simulink model "proportionalValveHarness"  (R2022b)
settings: Solver=VariableStepAuto  StartTime=0.0  StopTime=15  RelTol=1e-3  AbsTol=1e-3
libraries: fl_lib x6, nesl_utility x3, VentilatorLibrary x1
settings Model: Creator=agonzale  LastModifiedBy=fedformi_new
settings SolverCC: AutoScaleAbsTol=off  AlgebraicLoopSolver=TrustRegion
settings DebuggingCC: UnconnectedInputMsg=warning  UnconnectedOutputMsg=warning  UnconnectedLineMsg=warning  SymbolicDimsDataTypeCodeGenerationDiagnostic=none  SFMachineParentedDataDiag=warning
settings ModelReferenceCC: EnableRefExpFcnMdlSchedulingChecks=on
settings SFSimCC: CustomCodeUndefinedFunction=UseInterfaceOnly
settings SimscapeCC: SimscapeLogType=all  SimscapeLogSimulationStatistics=on  SimscapeLogLimitData=off  SimscapeLogDataHistory=10000

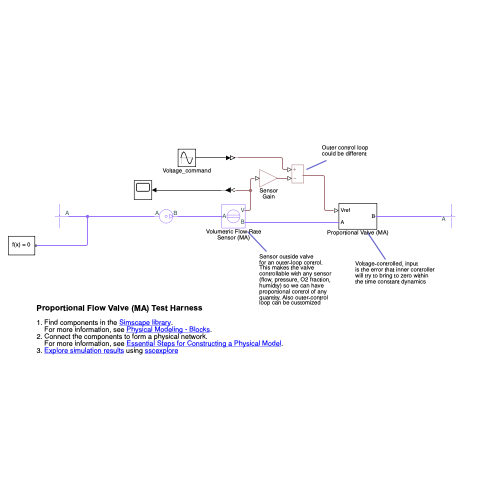
[thumbnail: Simulink's stored preview of the top-level diagram]
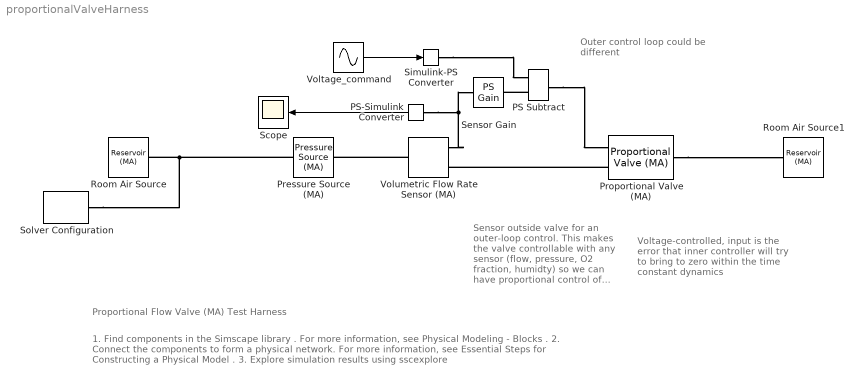
== system proportionalValveHarness ==
  note: Outer control loop
      | could be different
  note: Sensor outside valve
      | for an outer-loop control.
      | This makes the valve
      | controllable with any sensor
      | (flow, pressure, O2 fraction,
      | humidty) so we can have
      | proportional control of any
      | quantity. Also outer-control
      | loop can be customized
  note: Voltage-controlled, input
      | is the error that inner controller
      | will try to bring to zero within
      | the time constant dynamics
  note: 1. Find components in the Simscape library .
      | For more information, see Physical Modeling - Blocks .
      | 2. Connect the components to form a physical network.
      | For more information, see Essential Steps for Constructing a Physical Model .
      | 3. Explore simulation results using sscexplore
  note: Proportional Flow Valve (MA) Test Harness
  PS Subtract : fl_lib/Physical Signals/Functions/PS Subtract
  PS-Simulink Converter : nesl_utility/PS-Simulink Converter  PhysicalDomain=network_engine_domain  SubClassName=ps_output  LeftPortType=input  RightPortType=output  PseudoPeriodic=off  Frequencies=[]  VectorFormat=1-D array  Unit=lpm  AffineConversion=off
  Pressure Source (MA) : fl_lib/Moist Air/Sources/Pressure Source (MA)  power_spec=foundation.enum.power_spec.isentropic  pressure_differential=101 psi  area_A=pi*0.3^2/4 in^2  area_B=pi*0.3^2/4 in^2
      settings: InternalSimscapePortConfiguration="{\"Bottom\":[],\"Left\":[{\"id\":\"A\",\"label\":\"A\",\"type\":\"foundation.moist_air.moist_air\"}],\"Right\":[{\"id\":\"B\",\"label\":\"B\",\"type\":\"foundation.moist_air.moist_air\"}],\"Top\":[]}"
  Proportional Valve (MA) : VentilatorLibrary/Proportional Valve (MA)  D_max=0.125  area_leak=1e-5  area_A=pi*0.3^2/4  Cd=0.7  pr=0.999  area_init=1e-5  tau=0.1  Vmax=5
  Room Air Source : fl_lib/Moist Air/Elements/Reservoir (MA)  pressure_spec=foundation.enum.pressure_spec.atmospheric  reservoir_pressure=0.101325 MPa  temperature_spec=foundation.enum.temperature_spec.specified  reservoir_temperature=293 K  moisture_spec=foundation.enum.moisture_spec.relative_humidity  reservoir_RH=0.1  reservoir_x_w=0.01  reservoir_y_w=0.01  reservoir_HR=0.01  trace_gas_spec=foundation.enum.trace_gas_spec.mass_fraction  reservoir_x_g=0  reservoir_y_g=0.001  RH_ws=1  area_A=pi*0.3^2/4 in^2
  Room Air Source1 : fl_lib/Moist Air/Elements/Reservoir (MA)  pressure_spec=foundation.enum.pressure_spec.atmospheric  reservoir_pressure=0.101325 MPa  temperature_spec=foundation.enum.temperature_spec.specified  reservoir_temperature=25 degC  moisture_spec=foundation.enum.moisture_spec.relative_humidity  reservoir_RH=0.05  reservoir_x_w=0.01  reservoir_y_w=0.01  reservoir_HR=0.01  trace_gas_spec=foundation.enum.trace_gas_spec.mass_fraction  reservoir_x_g=0  reservoir_y_g=0.001  RH_ws=1  area_A=pi*0.3^2/4 in^2
  Scope : Scope
  Sensor Gain : fl_lib/Physical Signals/Functions/PS Gain  gain=5/500 V/lpm
  Simulink-PS Converter : nesl_utility/Simulink-PS Converter  PhysicalDomain=network_engine_domain  SubClassName=ps_input  LeftPortType=input  RightPortType=output  PseudoPeriodic=off  Frequencies=[]  NoiseDistribution=none  NoiseParameters=[]  Unit=V  AffineConversion=off  FilteringAndDerivatives=provide  SimscapeFilterOrder=1  InputFilterTimeConstant=0.001  UdotUserProvided=0
  Solver Configuration : nesl_utility/Solver Configuration  PhysicalDomain=network_engine_domain  SubClassName=solver  LeftPortType=input  RightPortType=generic  Tones=[]  Harmonics=[]  SimulateNoise=off  Profile=off  UseLocalSampling=off  EnableSwitchedLinearOptims=on  FrequencyDomain=off  UseCCode=off  RelTol=0.001  AbsTol=1e-06  MinStep=1e-09  ToWorkspace=off  RevertToSquareIcSolve=off  NumHomotopyIterations=100  PhasorMode=off  PhasorModeNumHarmonics=1  ConsistencySolver=NEWTON_XTOL_AFTER_FTOL  IndexReductionMethod=DerivativeReplacement  DoDC=off  ResidualTolerance=1e-09  ConsistencyTolSource=GLOBAL  ConsistencyAbsTol=0.001  ConsistencyRelTol=0.001  ConsistencyTolFactor=0.001  UseLocalSolver=off  LocalSolverChoice=NE_BACKWARD_EULER_ADVANCER  ResolveIndetEquations=on  FunctionEvalNumThread=1  LocalSolverSampleTime=1e-3  DoFixedCost=off  MaxNonlinIter=3  MaxModeIter=2  ComputeImpulses=off  ImpulseIterations=2  LinearAlgebra=auto  LinearAlgebraNumThread=0  EquationFormulation=NE_TIME_EF  DelaysMemoryBudget=1024  AutomaticFiltering=on  FilteringTimeConstant=0.001  PartitionStorageMethod=AS_NEEDED  PartitionMemoryBudget=1024  PartitionMethod=ROBUST
  Voltage_command : Sin  Amplitude=10  Frequency=2*pi/5  SampleTime=0
  Volumetric Flow Rate Sensor (MA) : fl_lib/Moist Air/Sensors/Volumetric Flow Rate Sensor (MA)  volumetric_flow_conditions=foundation.enum.volumetric_flow_conditions.standard  p_std=1 atm  T_std=293 K  RH_std=0.1
      settings: InternalSimscapePortConfiguration="{\"Bottom\":[],\"Left\":[{\"id\":\"A\",\"label\":\"A\",\"type\":\"foundation.moist_air.moist_air\"}],\"Right\":[{\"id\":\"B\",\"label\":\"B\",\"type\":\"foundation.moist_air.moist_air\"},{\"id\":\"V\",\"label\":\"V\",\"type\":\"output\"}],\"Top\":[]}"
  wires:
  Voltage_command/1 -> Simulink-PS Converter/1
  PS-Simulink Converter/1 -> Scope/1
  connections:
  Solver Configuration/RConn1 -- Pressure Source (MA)/LConn1 -- Room Air Source/LConn1
  Volumetric Flow Rate Sensor (MA)/RConn2 -- Sensor Gain/LConn1 -- PS-Simulink Converter/LConn1
  Proportional Valve (MA)/LConn2 -- Volumetric Flow Rate Sensor (MA)/RConn1
  PS Subtract/LConn2 -- Sensor Gain/RConn1
  PS Subtract/RConn1 -- Proportional Valve (MA)/LConn1
  Simulink-PS Converter/RConn1 -- PS Subtract/LConn1
  Volumetric Flow Rate Sensor (MA)/LConn1 -- Pressure Source (MA)/RConn1
  Proportional Valve (MA)/RConn1 -- Room Air Source1/LConn1
